simulink model "VITM"  (R2017b)
settings: Solver=FixedStepDiscrete  StartTime=0.0  StopTime=inf  FixedStep=vitk_stepSize  RelTol=1e-3  EnableMultiTasking=on
values from neighbouring files (symbols this model uses):
  vitc_CellPackVolTol = 12    [VITM_init.m]
  vitc_CellTempFaultTimer = 10    [VITM_init.m]
  vitc_CellTempFilterC = 1.0    (= 1)    [VITM_init.m]
  vitc_CellTempHighFaultReset = 0    [VITM_init.m]
  vitc_CellTempLowFaultReset = 0    [VITM_init.m]
  vitc_CellTempMax = 70    [VITM_init.m]
  vitc_CellTempMin = -40    [VITM_init.m]
  vitc_CellVolFilterC = 1    [VITM_init.m]
  vitc_CellVoltageFaultTimer = 2    [VITM_init.m]
  vitc_CellVoltageHighFaultReset = 0    [VITM_init.m]
  vitc_CellVoltageLowFaultReset = 0    [VITM_init.m]
  vitc_CellVoltageMax = 4.2    [VITM_init.m]
  vitc_CellVoltageMin = 2.7    [VITM_init.m]
  vitc_CoolantInletTFaultReset = 0    [VITM_init.m]
  vitc_CoolantInletTLowerLim = -40    [VITM_init.m]
  vitc_CoolantInletTUpperLim = 70    [VITM_init.m]
  vitc_CoolantOutletTFaultReset = 0    [VITM_init.m]
  vitc_CoolantOutletTLowerLim = -40    [VITM_init.m]
  vitc_CoolantOutletTUpperLim = 70    [VITM_init.m]
  vitc_CoolantTempFaultCounter = 5    [VITM_init.m]
  vitc_CoolantTFilterC = 0.9    [VITM_init.m]
  vitc_HVILFaultCounter = 1    [VITM_init.m]
  vitc_HVILFaultReset = 0    [VITM_init.m]
  vitc_PackCurFilterC = 1    [VITM_init.m]
  vitc_PackCurrentFaultReset = 0    [VITM_init.m]
  vitc_PackCurrentFaultTimer = 1    [VITM_init.m]
  vitc_PackCurrentLimit = 300    [VITM_init.m]
  vitc_PackVolFilterC = 1    [VITM_init.m]
  vitc_PackVoltageFaultReset = 0    [VITM_init.m]
  vitc_PackVoltageFaultTimer = 10    [VITM_init.m]
  vitc_VehVolFilterC = 1    [VITM_init.m]
  vitk_NumberInPara = 1    [VITM_init.m]
  vitk_NumberInSeries = 40    [VITM_init.m]
  vitk_stepSize = 0.1    [VITM_init.m]
libraries: simulink x1
settings Model: Creator=favv5g  LastModifiedBy=nctzv8
settings ConfigSet: Description=OpenECU configuration set for code generation under RTW-EC.
settings SolverCC: PositivePriorityOrder=on
settings DataIOCC: LimitDataPoints=on  SaveFormat=Array  SignalLogging=off  VisualizeSimOutput=off
settings OptimizationCC: DefaultParameterBehavior=Inlined  InlineInvariantSignals=on  ExpressionDepthLimit=2147483647  StateBitsets=on  DataBitsets=on  ZeroExternalMemoryAtStartup=off  ZeroInternalMemoryAtStartup=off  NoFixptDivByZeroProtection=on  EfficientFloat2IntCast=on  LifeSpan=1
settings DebuggingCC: SaveWithParameterizedLinksMsg=none  SignalResolutionControl=TryResolveAllWithWarning  MultiTaskDSMMsg=warning  MultiTaskCondExecSysMsg=none  SingleTaskRateTransMsg=error  CheckMatrixSingularityMsg=warning  VectorMatrixConversionMsg=warning  FcnCallInpInsideContextMsg=warning  SignalLabelMismatchMsg=warning  AllowSymbolicDim=off  StateNameClashWarn=warning  SFUnexpectedBacktrackingDiag=warning  SFNoUnconditionalDefaultTransitionDiag=warning  SFExecutionAtInitializationDiag=none
settings HardwareCC: ProdBitPerPointer=32  ProdBitPerSizeT=32  ProdBitPerPtrDiffT=32  ProdLargestAtomicInteger=Long  ProdLargestAtomicFloat=Double  ProdEndianess=BigEndian  ProdWordSize=32  ProdHWDeviceType=Freescale->32-bit PowerPC  TargetIntDivRoundTo=Zero  TargetEndianess=BigEndian  TargetHWDeviceType=Freescale->32-bit PowerPC  ProdEqTarget=off
settings ModelReferenceCC: PropagateSignalLabelsOutOfModel=off
settings SFSimCC: MATLABDynamicMemAlloc=off
settings RTWCC: SystemTargetFile=openecu_ert.tlc  MakeCommand=make_rtw optimized_floating_point=1  TemplateMakefile=openecu_ert_r2015b_64.tmf  Description=OpenECU Platform Target (ERT, optimised floating-point code)  RetainRTWFile=on  IncludeHyperlinkInReport=on
settings CodeAppCC: ForceParamTrailComments=on  IgnoreCustomStorageClasses=off  SimulinkDataObjDesc=on  CustomSymbolStrType=$N$R$M  InsertBlockDesc=on  StateflowObjectComments=on  InternalIdentifier=Classic
settings STFCustomTargetCC: TargetLibSuffix=.a  GenerateSampleERTMain=on  IncludeMdlTerminateFcn=off  CombineOutputUpdateFcns=on  IncludeFileDelimiter=UseQuote  ERTCustomFileBanners=on  SupportContinuousTime=off  RemoveResetFunc=on  MATLABClassNameForMDSCustomization=Simulink.SoftwareTarget.ERTCustomization  GRTInterface=off  SystemTargetFile=openecu_ert.tlc
settings ERTTargetCC: MultiwordLength=2048  GenerateSampleERTMain=on  ParMdlRefBuildCompliant=off  CompOptLevelCompliant=off  ConcurrentExecutionCompliant=off  IncludeMdlTerminateFcn=off  IncludeFileDelimiter=UseQuote  SupportNonInlinedSFcns=on  ModelStepFunctionPrototypeControlCompliant=off  CPPClassGenCompliant=off  UseToolchainInfoCompliant=off  ExtModeMexFile=noextcomm  InlinedParameterPlacement=NonHierarchical  ERTSrcFileBannerTemplate=oe_code_c_template.cgt  ERTHdrFileBannerTemplate=oe_code_h_template.cgt  ERTDataSrcFileTemplate=oe_data_c_template.cgt  ERTDataHdrFileTemplate=oe_data_h_template.cgt  ERTCustomFileTemplate=example_file_process.tlc  GlobalDataDefinition=InSeparateSourceFile  GlobalDataReference=InSeparateHeaderFile  ConvertIfToSwitch=off  SuppressUnreachableDefaultCases=off  EnableUserReplacementTypes=on
settings ConfigComp: CovMetricSettings=dw  CovHtmlReporting=on  CovSaveCumulativeToWorkspaceVar=on  CovSaveSingleToWorkspaceVar=on  CovExternalEMLEnable=off

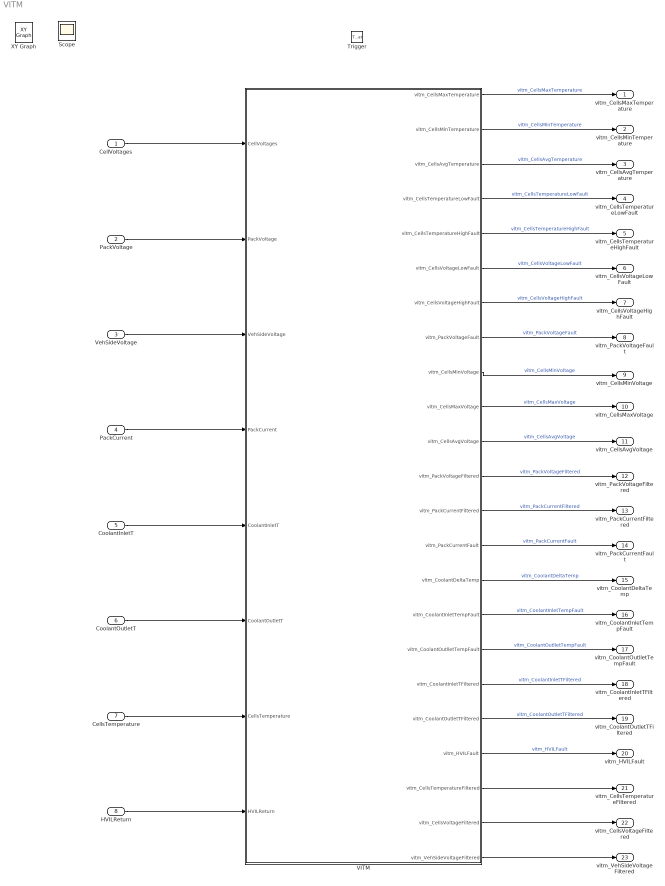
== system VITM ==
  CellVoltages : Inport  PortDimensions=40
  PackVoltage : Inport  Port=2
  VehSideVoltage : Inport  Port=3
  PackCurrent : Inport  Port=4
  CoolantInletT : Inport  Port=5
  CoolantOutletT : Inport  Port=6
  CellsTemperature : Inport  Port=7  PortDimensions=40
  HVILReturn : Inport  Port=8
  Trigger : TriggerPort  TriggerType=function-call  VariantControl=(inherit)  PortDimensions=1
  VITM : Subsystem  TreatAsAtomicUnit=on
  vitm_CellsMaxTemperature : Outport
  vitm_CellsMinTemperature : Outport  Port=2
  vitm_CellsAvgTemperature : Outport  Port=3
  vitm_CellsTemperatureLowFault : Outport  Port=4
  vitm_CellsTemperatureHighFault : Outport  Port=5
  vitm_CellsVoltageLowFault : Outport  Port=6
  vitm_CellsVoltageHighFault : Outport  Port=7
  vitm_PackVoltageFault : Outport  Port=8
  vitm_CellsMinVoltage : Outport  Port=9
  vitm_CellsMaxVoltage : Outport  Port=10
  vitm_CellsAvgVoltage : Outport  Port=11
  vitm_PackVoltageFiltered : Outport  Port=12
  vitm_PackCurrentFiltered : Outport  Port=13
  vitm_PackCurrentFault : Outport  Port=14
  vitm_CoolantDeltaTemp : Outport  Port=15
  vitm_CoolantInletTempFault : Outport  Port=16
  vitm_CoolantOutlletTempFault : Outport  Port=17
  vitm_CoolantInletTFiltered : Outport  Port=18
  vitm_CoolantOutletTFiltered : Outport  Port=19
  vitm_HVILFault : Outport  Port=20
  vitm_CellsTemperatureFiltered : Outport  Port=21
  vitm_CellsVoltageFiltered : Outport  Port=22  PortDimensions=40
  vitm_VehSideVoltageFiltered : Outport  Port=23
  Scope : Scope
  XY Graph : simulink/Sinks/XY Graph  IOType=viewer  xmin=-1  xmax=1  ymin=-1  ymax=1  st=-1
  wires:
  CellVoltages/1 -> VITM/1(CellVoltages)
  PackVoltage/1 -> VITM/2(PackVoltage)
  VehSideVoltage/1 -> VITM/3(VehSideVoltage)
  PackCurrent/1 -> VITM/4(PackCurrent)
  CoolantInletT/1 -> VITM/5(CoolantInletT)
  CoolantOutletT/1 -> VITM/6(CoolantOutletT)
  CellsTemperature/1 -> VITM/7(CellsTemperature)
  VITM/2(vitm_CellsMinTemperature) -> vitm_CellsMinTemperature/1  "vitm_CellsMinTemperature"
  VITM/3(vitm_CellsAvgTemperature) -> vitm_CellsAvgTemperature/1  "vitm_CellsAvgTemperature"
  VITM/1(vitm_CellsMaxTemperature) -> vitm_CellsMaxTemperature/1  "vitm_CellsMaxTemperature"
  VITM/4(vitm_CellsTemperatureLowFault) -> vitm_CellsTemperatureLowFault/1  "vitm_CellsTemperatureLowFault"
  VITM/6(vitm_CellsVoltageLowFault) -> vitm_CellsVoltageLowFault/1  "vitm_CellsVoltageLowFault"
  VITM/7(vitm_CellsVoltageHighFault) -> vitm_CellsVoltageHighFault/1  "vitm_CellsVoltageHighFault"
  VITM/5(vitm_CellsTemperatureHighFault) -> vitm_CellsTemperatureHighFault/1  "vitm_CellsTemperatureHighFault"
  VITM/9(vitm_CellsMinVoltage) -> vitm_CellsMinVoltage/1  "vitm_CellsMinVoltage"
  VITM/8(vitm_PackVoltageFault) -> vitm_PackVoltageFault/1  "vitm_PackVoltageFault"
  VITM/18(vitm_CoolantInletTFiltered) -> vitm_CoolantInletTFiltered/1  "vitm_CoolantInletTFiltered"
  VITM/10(vitm_CellsMaxVoltage) -> vitm_CellsMaxVoltage/1  "vitm_CellsMaxVoltage"
  VITM/12(vitm_PackVoltageFiltered) -> vitm_PackVoltageFiltered/1  "vitm_PackVoltageFiltered"
  VITM/14(vitm_PackCurrentFault) -> vitm_PackCurrentFault/1  "vitm_PackCurrentFault"
  VITM/15(vitm_CoolantDeltaTemp) -> vitm_CoolantDeltaTemp/1  "vitm_CoolantDeltaTemp"
  VITM/13(vitm_PackCurrentFiltered) -> vitm_PackCurrentFiltered/1  "vitm_PackCurrentFiltered"
  VITM/11(vitm_CellsAvgVoltage) -> vitm_CellsAvgVoltage/1  "vitm_CellsAvgVoltage"
  VITM/16(vitm_CoolantInletTempFault) -> vitm_CoolantInletTempFault/1  "vitm_CoolantInletTempFault"
  VITM/17(vitm_CoolantOutlletTempFault) -> vitm_CoolantOutlletTempFault/1  "vitm_CoolantOutlletTempFault"
  VITM/19(vitm_CoolantOutletTFiltered) -> vitm_CoolantOutletTFiltered/1  "vitm_CoolantOutletTFiltered"
  HVILReturn/1 -> VITM/8(HVILReturn)
  VITM/23(vitm_VehSideVoltageFiltered) -> vitm_VehSideVoltageFiltered/1
  VITM/22(vitm_CellsVoltageFiltered) -> vitm_CellsVoltageFiltered/1
  VITM/21(vitm_CellsTemperatureFiltered) -> vitm_CellsTemperatureFiltered/1
  VITM/20(vitm_HVILFault) -> vitm_HVILFault/1  "vitm_HVILFault"

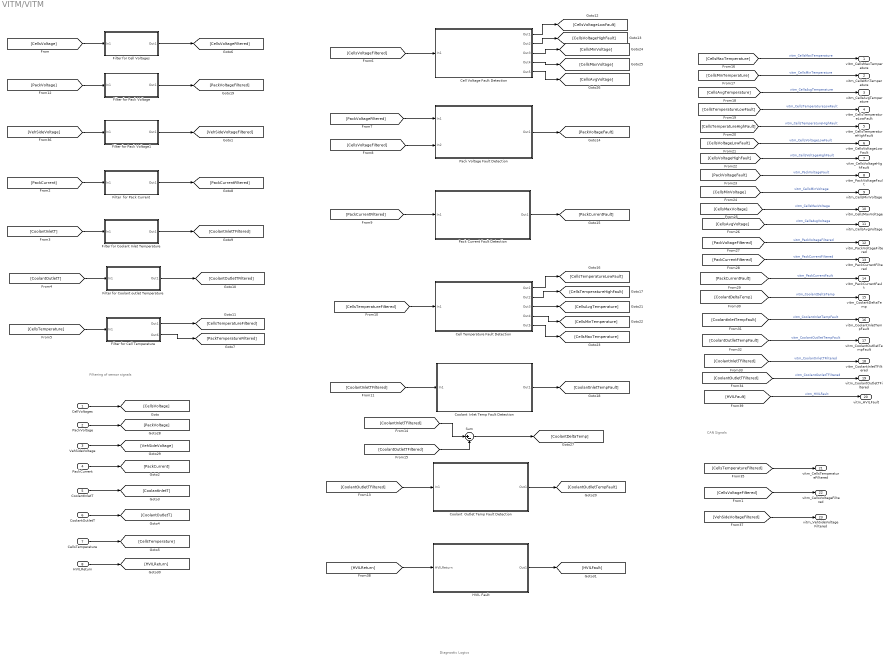
== system VITM/VITM ==
  note: Diagnostic Logics
  note: Filtering of sensor signals
  note: CAN Signals
  CellVoltages : Inport  PortDimensions=40
  PackVoltage : Inport  Port=2
  VehSideVoltage : Inport  Port=3
  PackCurrent : Inport  Port=4
  CoolantInletT : Inport  Port=5
  CoolantOutletT : Inport  Port=6
  CellsTemperature : Inport  Port=7  PortDimensions=40
  HVILReturn : Inport  Port=8
  " Filter for Cell Voltages" : Subsystem
  " Filter for Pack Voltage" : Subsystem
  " Filter for Pack Voltage1" : Subsystem
  Cell Temperature Fault Detection : Subsystem
  Cell Voltage Fault Detection : Subsystem
  Coolant  Inlet Temp Fault Detection : Subsystem
  Coolant  Outlet Temp Fault Detection : Subsystem
  Filter  for Pack Current : Subsystem
  Filter for Cell Temperature : Subsystem
  Filter for Coolant Inlet Temperature : Subsystem
  Filter for Coolant outlet Temperature : Subsystem
  HVIL Fault : Subsystem
  Pack Current Fault Detection : Subsystem
  Pack Voltage Fault Detection : Subsystem
  Sum : Sum  Inputs=|+-
  vitm_CellsMaxTemperature : Outport
  vitm_CellsMinTemperature : Outport  Port=2
  vitm_CellsAvgTemperature : Outport  Port=3
  vitm_CellsTemperatureLowFault : Outport  Port=4
  vitm_CellsTemperatureHighFault : Outport  Port=5
  vitm_CellsVoltageLowFault : Outport  Port=6
  vitm_CellsVoltageHighFault : Outport  Port=7
  vitm_PackVoltageFault : Outport  Port=8
  vitm_CellsMinVoltage : Outport  Port=9
  vitm_CellsMaxVoltage : Outport  Port=10
  vitm_CellsAvgVoltage : Outport  Port=11
  vitm_PackVoltageFiltered : Outport  Port=12
  vitm_PackCurrentFiltered : Outport  Port=13
  vitm_PackCurrentFault : Outport  Port=14
  vitm_CoolantDeltaTemp : Outport  Port=15
  vitm_CoolantInletTempFault : Outport  Port=16
  vitm_CoolantOutlletTempFault : Outport  Port=17
  vitm_CoolantInletTFiltered : Outport  Port=18
  vitm_CoolantOutletTFiltered : Outport  Port=19
  vitm_HVILFault : Outport  Port=20
  vitm_CellsTemperatureFiltered : Outport  Port=21
  vitm_CellsVoltageFiltered : Outport  Port=22
  vitm_VehSideVoltageFiltered : Outport  Port=23
  wires:
  [VehSideVoltage] -> " Filter for Pack Voltage1"/1(In1)
  VehSideVoltage/1 -> [VehSideVoltage]
  " Filter for Pack Voltage1"/1(Out1) -> [VehSideVoltageFiltered]
  [VehSideVoltageFiltered] -> vitm_VehSideVoltageFiltered/1
  [PackVoltage] -> " Filter for Pack Voltage"/1(In1)
  PackVoltage/1 -> [PackVoltage]
  " Filter for Pack Voltage"/1(Out1) -> [PackVoltageFiltered]
  CoolantOutletT/1 -> [CoolantOutletT]
  Filter  for Pack Current/1(Out1) -> [PackCurrentFiltered]
  [CoolantInletT] -> Filter for Coolant Inlet Temperature/1(In1)
  Filter for Coolant Inlet Temperature/1(Out1) -> [CoolantInletTFiltered]
  [CellsVoltage] -> " Filter for Cell Voltages"/1(In1)
  CellVoltages/1 -> [CellsVoltage]
  PackCurrent/1 -> [PackCurrent]
  CellsTemperature/1 -> [CellsTemperature]
  CoolantInletT/1 -> [CoolantInletT]
  " Filter for Cell Voltages"/1(Out1) -> [CellsVoltageFiltered]
  [PackCurrent] -> Filter  for Pack Current/1(In1)
  Cell Voltage Fault Detection/2(Out2) -> [CellsVoltageHighFault]
  Pack Current Fault Detection/1(Out1) -> [PackCurrentFault]
  [CoolantOutletT] -> Filter for Coolant outlet Temperature/1(In1)
  [CellsTemperatureFiltered] -> Cell Temperature Fault Detection/1(In1)
  Cell Temperature Fault Detection/2(Out2) -> [CellsTemperatureHighFault]
  Coolant  Inlet Temp Fault Detection/1(Out1) -> [CoolantInletTempFault]
  [CellsTemperature] -> Filter for Cell Temperature/1(In1)
  [PackVoltageFiltered] -> Pack Voltage Fault Detection/1(In1)
  Cell Temperature Fault Detection/1(Out1) -> [CellsTemperatureLowFault]
  Cell Voltage Fault Detection/1(Out1) -> [CellsVoltageLowFault]
  Cell Temperature Fault Detection/5(Out5) -> [CellsMaxTemperature]
  Cell Temperature Fault Detection/4(Out4) -> [CellsMinTemperature]
  Cell Voltage Fault Detection/3(Out3) -> [CellsMinVoltage]
  [CellsVoltageFiltered] -> Pack Voltage Fault Detection/2(In2)
  Cell Voltage Fault Detection/4(Out4) -> [CellsMaxVoltage]
  [CoolantInletTFiltered] -> Sum/1
  [CellsVoltageFiltered] -> Cell Voltage Fault Detection/1(In1)
  [PackCurrentFiltered] -> Pack Current Fault Detection/1(In1)
  [CoolantOutletTFiltered] -> Sum/2
  Sum/1 -> [CoolantDeltaTemp]
  [CellsMinTemperature] -> vitm_CellsMinTemperature/1  "vitm_CellsMinTemperature"
  [CoolantInletTFiltered] -> Coolant  Inlet Temp Fault Detection/1(In1)
  [CellsAvgTemperature] -> vitm_CellsAvgTemperature/1  "vitm_CellsAvgTemperature"
  Coolant  Outlet Temp Fault Detection/1(Out1) -> [CoolantOutlletTempFault]
  [CoolantOutletTFiltered] -> Coolant  Outlet Temp Fault Detection/1(In1)
  Cell Voltage Fault Detection/5(Out5) -> [CellsAvgVoltage]
  Cell Temperature Fault Detection/3(Out3) -> [CellsAvgTemperature]
  [CellsMaxTemperature] -> vitm_CellsMaxTemperature/1  "vitm_CellsMaxTemperature"
  Filter for Cell Temperature/1(Out1) -> [CellsTemperatureFiltered]
  Filter for Coolant outlet Temperature/1(Out1) -> [CoolantOutletTFiltered]
  Pack Voltage Fault Detection/1(Out1) -> [PackVoltageFault]
  [CellsTemperatureLowFault] -> vitm_CellsTemperatureLowFault/1  "vitm_CellsTemperatureLowFault"
  [CellsVoltageLowFault] -> vitm_CellsVoltageLowFault/1  "vitm_CellsVoltageLowFault"
  [CellsVoltageHighFault] -> vitm_CellsVoltageHighFault/1  "vitm_CellsVoltageHighFault"
  [CellsTemperatureHighFault] -> vitm_CellsTemperatureHighFault/1  "vitm_CellsTemperatureHighFault"
  [CellsMinVoltage] -> vitm_CellsMinVoltage/1  "vitm_CellsMinVoltage"
  [PackVoltageFault] -> vitm_PackVoltageFault/1  "vitm_PackVoltageFault"
  [CoolantInletTFiltered] -> vitm_CoolantInletTFiltered/1  "vitm_CoolantInletTFiltered"
  [CellsMaxVoltage] -> vitm_CellsMaxVoltage/1  "vitm_CellsMaxVoltage"
  [PackVoltageFiltered] -> vitm_PackVoltageFiltered/1  "vitm_PackVoltageFiltered"
  [PackCurrentFault] -> vitm_PackCurrentFault/1  "vitm_PackCurrentFault"
  [CoolantDeltaTemp] -> vitm_CoolantDeltaTemp/1  "vitm_CoolantDeltaTemp"
  [PackCurrentFiltered] -> vitm_PackCurrentFiltered/1  "vitm_PackCurrentFiltered"
  [CellsAvgVoltage] -> vitm_CellsAvgVoltage/1  "vitm_CellsAvgVoltage"
  [CoolantInletTempFault] -> vitm_CoolantInletTempFault/1  "vitm_CoolantInletTempFault"
  [CoolantOutlletTempFault] -> vitm_CoolantOutlletTempFault/1  "vitm_CoolantOutlletTempFault"
  [CoolantOutletTFiltered] -> vitm_CoolantOutletTFiltered/1  "vitm_CoolantOutletTFiltered"
  Filter for Cell Temperature/2(Out6) -> [PackTemperatureFiltered]
  [CellsTemperatureFiltered] -> vitm_CellsTemperatureFiltered/1
  [CellsVoltageFiltered] -> vitm_CellsVoltageFiltered/1
  HVILReturn/1 -> [HVILReturn]
  HVIL Fault/1(Out1) -> [HVILFault]
  [HVILReturn] -> HVIL Fault/1(HVILReturn)
  [HVILFault] -> vitm_HVILFault/1  "vitm_HVILFault"

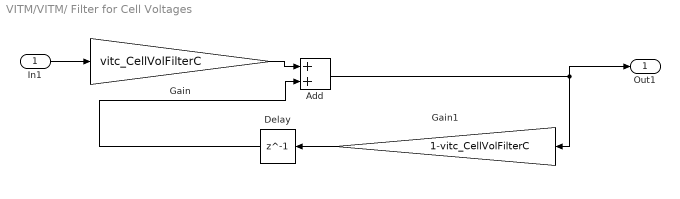
== system VITM/VITM/ Filter for Cell Voltages ==
  In1 : Inport
  Add : Sum
  Delay : Delay  DelayLength=1
  Gain : Gain  Gain=vitc_CellVolFilterC
  Gain1 : Gain  Gain=1-vitc_CellVolFilterC
  Out1 : Outport
  wires:
  Add/1 -> Out1/1, Gain1/1
  Gain1/1 -> Delay/1
  Delay/1 -> Add/2
  In1/1 -> Gain/1
  Gain/1 -> Add/1

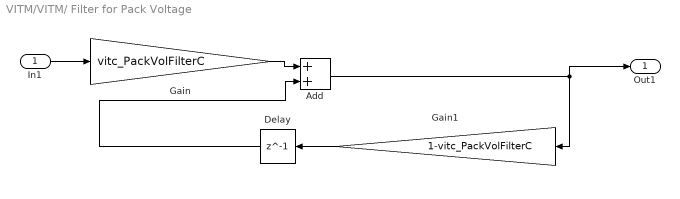
== system VITM/VITM/ Filter for Pack Voltage ==
  In1 : Inport
  Add : Sum
  Delay : Delay  DelayLength=1
  Gain : Gain  Gain=vitc_PackVolFilterC
  Gain1 : Gain  Gain=1-vitc_PackVolFilterC
  Out1 : Outport
  wires:
  Add/1 -> Out1/1, Gain1/1
  Gain1/1 -> Delay/1
  Delay/1 -> Add/2
  In1/1 -> Gain/1
  Gain/1 -> Add/1

== system VITM/VITM/ Filter for Pack Voltage1 ==
  In1 : Inport
  Add : Sum
  Delay : Delay  DelayLength=1
  Gain : Gain  Gain=vitc_VehVolFilterC
  Gain1 : Gain  Gain=1-vitc_VehVolFilterC
  Out1 : Outport
  wires:
  Add/1 -> Out1/1, Gain1/1
  Gain1/1 -> Delay/1
  Delay/1 -> Add/2
  In1/1 -> Gain/1
  Gain/1 -> Add/1

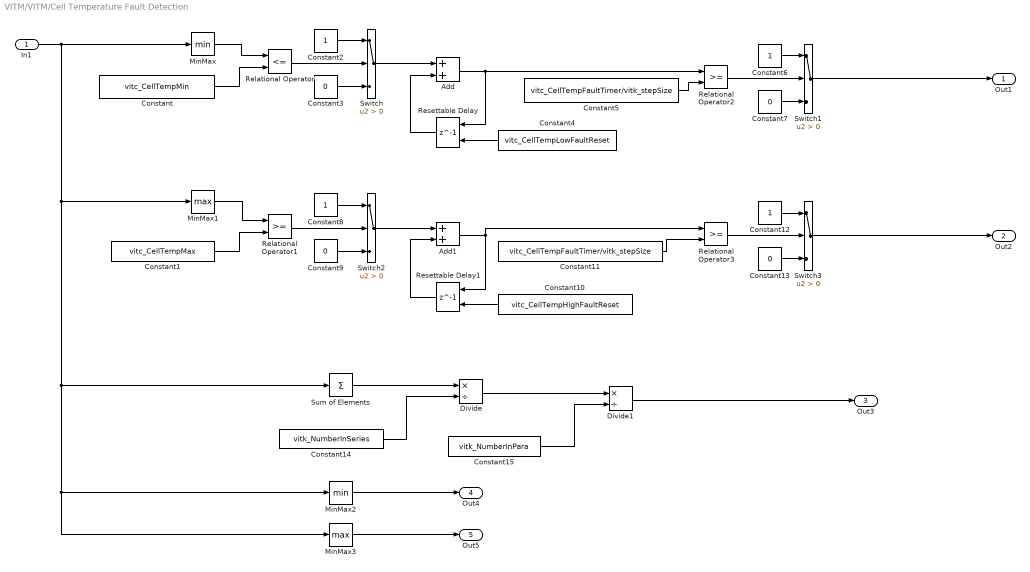
== system VITM/VITM/Cell Temperature Fault Detection ==
  In1 : Inport
  Add : Sum
  Add1 : Sum
  Constant : Constant  Value=vitc_CellTempMin
  Constant1 : Constant  Value=vitc_CellTempMax
  Constant10 : Constant  Value=vitc_CellTempHighFaultReset
  Constant11 : Constant  Value=vitc_CellTempFaultTimer/vitk_stepSize
  Constant12 : Constant  OutDataTypeStr=uint8
  Constant13 : Constant  Value=0  OutDataTypeStr=uint8
  Constant14 : Constant  Value=vitk_NumberInSeries
  Constant15 : Constant  Value=vitk_NumberInPara
  Constant2 : Constant
  Constant3 : Constant  Value=0
  Constant4 : Constant  Value=vitc_CellTempLowFaultReset
  Constant5 : Constant  Value=vitc_CellTempFaultTimer/vitk_stepSize
  Constant6 : Constant  OutDataTypeStr=uint8
  Constant7 : Constant  Value=0  OutDataTypeStr=uint8
  Constant8 : Constant
  Constant9 : Constant  Value=0
  Divide : Product  Inputs=*/
  Divide1 : Product  Inputs=*/
  MinMax : MinMax
  MinMax1 : MinMax  Function=max
  MinMax2 : MinMax
  MinMax3 : MinMax  Function=max
  Relational Operator : RelationalOperator  Operator=<=  OutDataTypeStr=boolean  RndMeth=Nearest
  Relational Operator1 : RelationalOperator  OutDataTypeStr=boolean  RndMeth=Nearest
  Relational Operator2 : RelationalOperator  OutDataTypeStr=boolean  RndMeth=Nearest
  Relational Operator3 : RelationalOperator  OutDataTypeStr=boolean  RndMeth=Nearest
  Resettable Delay : Delay  DelayLength=1  ExternalReset=Rising
      settings: InputPortMap=u0,r5
  Resettable Delay1 : Delay  DelayLength=1  ExternalReset=Rising
      settings: InputPortMap=u0,r5
  Sum of Elements : Sum  Inputs=+
  Switch{,1..3} (4 alike) : Switch  Criteria=u2 > Threshold
  Out1 : Outport
  Out2 : Outport  Port=2
  Out3 : Outport  Port=3
  Out4 : Outport  Port=4
  Out5 : Outport  Port=5
  wires:
  Constant4/1 -> Resettable Delay/2
  Constant3/1 -> Switch/3
  Relational Operator/1 -> Switch/2
  Relational Operator2/1 -> Switch1/2
  Constant2/1 -> Switch/1
  Constant6/1 -> Switch1/1
  Constant7/1 -> Switch1/3
  MinMax/1 -> Relational Operator/1
  Constant/1 -> Relational Operator/2
  MinMax1/1 -> Relational Operator1/1
  Constant1/1 -> Relational Operator1/2
  Switch3/1 -> Out2/1
  Switch1/1 -> Out1/1
  Switch/1 -> Add/1
  Add/1 -> Relational Operator2/1, Resettable Delay/1
  Constant5/1 -> Relational Operator2/2
  Resettable Delay/1 -> Add/2
  Add1/1 -> Relational Operator3/1, Resettable Delay1/1
  Constant9/1 -> Switch2/3
  Constant8/1 -> Switch2/1
  Constant11/1 -> Relational Operator3/2
  Constant10/1 -> Resettable Delay1/2
  Constant13/1 -> Switch3/3
  Constant12/1 -> Switch3/1
  Switch2/1 -> Add1/1
  Relational Operator3/1 -> Switch3/2
  Relational Operator1/1 -> Switch2/2
  Resettable Delay1/1 -> Add1/2
  In1/1 -> MinMax/1, MinMax1/1, Sum of Elements/1, MinMax2/1, MinMax3/1
  Sum of Elements/1 -> Divide/1
  Constant14/1 -> Divide/2
  Divide/1 -> Divide1/1
  Constant15/1 -> Divide1/2
  Divide1/1 -> Out3/1
  MinMax2/1 -> Out4/1
  MinMax3/1 -> Out5/1

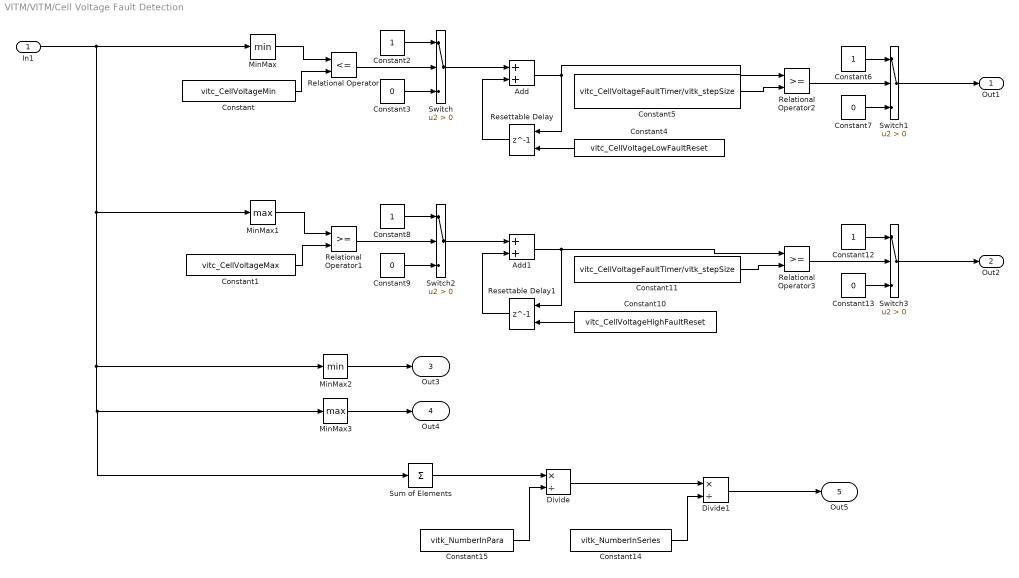
== system VITM/VITM/Cell Voltage Fault Detection ==
  In1 : Inport
  Add : Sum
  Add1 : Sum
  Constant : Constant  Value=vitc_CellVoltageMin
  Constant1 : Constant  Value=vitc_CellVoltageMax
  Constant10 : Constant  Value=vitc_CellVoltageHighFaultReset
  Constant11 : Constant  Value=vitc_CellVoltageFaultTimer/vitk_stepSize
  Constant12 : Constant  OutDataTypeStr=uint8
  Constant13 : Constant  Value=0  OutDataTypeStr=uint8
  Constant14 : Constant  Value=vitk_NumberInSeries
  Constant15 : Constant  Value=vitk_NumberInPara
  Constant2 : Constant
  Constant3 : Constant  Value=0
  Constant4 : Constant  Value=vitc_CellVoltageLowFaultReset
  Constant5 : Constant  Value=vitc_CellVoltageFaultTimer/vitk_stepSize
  Constant6 : Constant  OutDataTypeStr=uint8
  Constant7 : Constant  Value=0  OutDataTypeStr=uint8
  Constant8 : Constant
  Constant9 : Constant  Value=0
  Divide : Product  Inputs=*/
  Divide1 : Product  Inputs=*/  OutDataTypeStr=double
  MinMax : MinMax
  MinMax1 : MinMax  Function=max
  MinMax2 : MinMax
  MinMax3 : MinMax  Function=max
  Relational Operator : RelationalOperator  Operator=<=  OutDataTypeStr=boolean  RndMeth=Nearest
  Relational Operator1 : RelationalOperator  OutDataTypeStr=boolean  RndMeth=Nearest
  Relational Operator2 : RelationalOperator  OutDataTypeStr=boolean  RndMeth=Nearest
  Relational Operator3 : RelationalOperator  OutDataTypeStr=boolean  RndMeth=Nearest
  Resettable Delay : Delay  DelayLength=1  ExternalReset=Rising
      settings: InputPortMap=u0,r5
  Resettable Delay1 : Delay  DelayLength=1  ExternalReset=Rising
      settings: InputPortMap=u0,r5
  Sum of Elements : Sum  Inputs=+
  Switch{,1..3} (4 alike) : Switch  Criteria=u2 > Threshold
  Out1 : Outport
  Out2 : Outport  Port=2
  Out3 : Outport  Port=3
  Out4 : Outport  Port=4
  Out5 : Outport  Port=5  OutDataTypeStr=double
  wires:
  Constant4/1 -> Resettable Delay/2
  Constant3/1 -> Switch/3
  Relational Operator/1 -> Switch/2
  Relational Operator2/1 -> Switch1/2
  Constant2/1 -> Switch/1
  Constant6/1 -> Switch1/1
  Constant7/1 -> Switch1/3
  MinMax/1 -> Relational Operator/1
  Constant/1 -> Relational Operator/2
  MinMax1/1 -> Relational Operator1/1
  Constant1/1 -> Relational Operator1/2
  Switch3/1 -> Out2/1
  Switch1/1 -> Out1/1
  Switch/1 -> Add/1
  Add/1 -> Relational Operator2/1, Resettable Delay/1
  Constant5/1 -> Relational Operator2/2
  Resettable Delay/1 -> Add/2
  Add1/1 -> Relational Operator3/1, Resettable Delay1/1
  Constant9/1 -> Switch2/3
  Constant8/1 -> Switch2/1
  Constant11/1 -> Relational Operator3/2
  Constant10/1 -> Resettable Delay1/2
  Constant13/1 -> Switch3/3
  Constant12/1 -> Switch3/1
  Switch2/1 -> Add1/1
  Relational Operator3/1 -> Switch3/2
  Relational Operator1/1 -> Switch2/2
  Resettable Delay1/1 -> Add1/2
  MinMax2/1 -> Out3/1
  MinMax3/1 -> Out4/1
  In1/1 -> MinMax/1, MinMax1/1, MinMax2/1, MinMax3/1, Sum of Elements/1
  Sum of Elements/1 -> Divide/1
  Divide/1 -> Divide1/1
  Divide1/1 -> Out5/1
  Constant15/1 -> Divide/2
  Constant14/1 -> Divide1/2

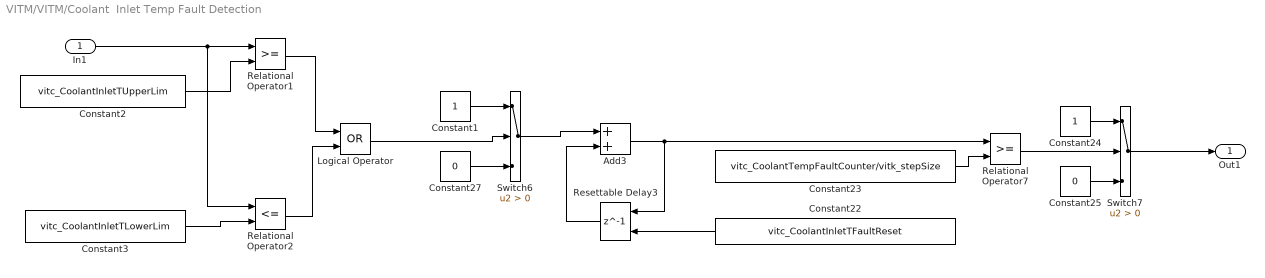
== system VITM/VITM/Coolant  Inlet Temp Fault Detection ==
  In1 : Inport
  Add3 : Sum
  Constant1 : Constant
  Constant2 : Constant  Value=vitc_CoolantInletTUpperLim
  Constant22 : Constant  Value=vitc_CoolantInletTFaultReset
  Constant23 : Constant  Value=vitc_CoolantTempFaultCounter/vitk_stepSize
  Constant24 : Constant  OutDataTypeStr=uint8
  Constant25 : Constant  Value=0  OutDataTypeStr=uint8
  Constant27 : Constant  Value=0
  Constant3 : Constant  Value=vitc_CoolantInletTLowerLim
  Logical Operator : Logic  Operator=OR  AllPortsSameDT=off  OutDataTypeStr=boolean
  Relational Operator1 : RelationalOperator  OutDataTypeStr=boolean  RndMeth=Nearest
  Relational Operator2 : RelationalOperator  Operator=<=  OutDataTypeStr=boolean  RndMeth=Nearest
  Relational Operator7 : RelationalOperator  OutDataTypeStr=boolean  RndMeth=Nearest
  Resettable Delay3 : Delay  DelayLength=1  ExternalReset=Rising
      settings: InputPortMap=u0,r5
  Switch6 : Switch  Criteria=u2 > Threshold
  Switch7 : Switch  Criteria=u2 > Threshold
  Out1 : Outport
  wires:
  Constant25/1 -> Switch7/3
  Constant27/1 -> Switch6/3
  Constant23/1 -> Relational Operator7/2
  Switch6/1 -> Add3/1
  Constant1/1 -> Switch6/1
  Constant24/1 -> Switch7/1
  Constant22/1 -> Resettable Delay3/2
  Add3/1 -> Relational Operator7/1, Resettable Delay3/1
  Resettable Delay3/1 -> Add3/2
  Switch7/1 -> Out1/1
  Relational Operator7/1 -> Switch7/2
  Constant2/1 -> Relational Operator1/2
  Constant3/1 -> Relational Operator2/2
  Relational Operator1/1 -> Logical Operator/1
  Relational Operator2/1 -> Logical Operator/2
  Logical Operator/1 -> Switch6/2
  In1/1 -> Relational Operator2/1, Relational Operator1/1

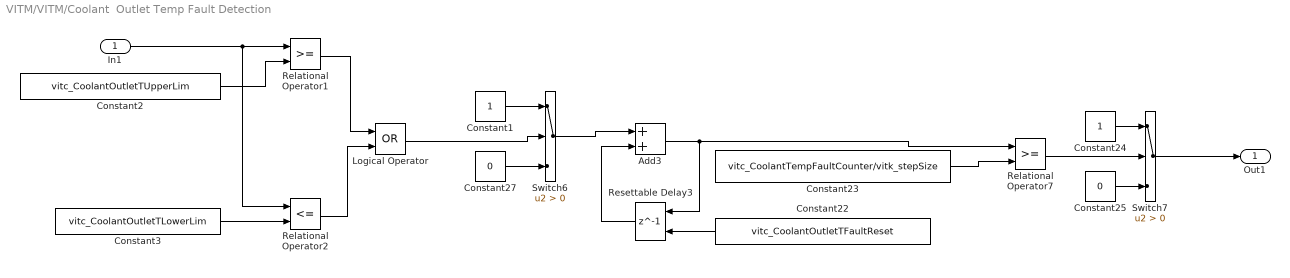
== system VITM/VITM/Coolant  Outlet Temp Fault Detection ==
  In1 : Inport
  Add3 : Sum
  Constant1 : Constant
  Constant2 : Constant  Value=vitc_CoolantOutletTUpperLim
  Constant22 : Constant  Value=vitc_CoolantOutletTFaultReset
  Constant23 : Constant  Value=vitc_CoolantTempFaultCounter/vitk_stepSize
  Constant24 : Constant  OutDataTypeStr=uint8
  Constant25 : Constant  Value=0  OutDataTypeStr=uint8
  Constant27 : Constant  Value=0
  Constant3 : Constant  Value=vitc_CoolantOutletTLowerLim
  Logical Operator : Logic  Operator=OR  AllPortsSameDT=off  OutDataTypeStr=boolean
  Relational Operator1 : RelationalOperator  OutDataTypeStr=boolean  RndMeth=Nearest
  Relational Operator2 : RelationalOperator  Operator=<=  OutDataTypeStr=boolean  RndMeth=Nearest
  Relational Operator7 : RelationalOperator  OutDataTypeStr=boolean  RndMeth=Nearest
  Resettable Delay3 : Delay  DelayLength=1  ExternalReset=Rising
      settings: InputPortMap=u0,r5
  Switch6 : Switch  Criteria=u2 > Threshold
  Switch7 : Switch  Criteria=u2 > Threshold
  Out1 : Outport
  wires:
  Constant25/1 -> Switch7/3
  Constant27/1 -> Switch6/3
  Constant23/1 -> Relational Operator7/2
  Switch6/1 -> Add3/1
  Constant1/1 -> Switch6/1
  Constant24/1 -> Switch7/1
  Constant22/1 -> Resettable Delay3/2
  Add3/1 -> Relational Operator7/1, Resettable Delay3/1
  Resettable Delay3/1 -> Add3/2
  Switch7/1 -> Out1/1
  Relational Operator7/1 -> Switch7/2
  In1/1 -> Relational Operator2/1, Relational Operator1/1
  Constant2/1 -> Relational Operator1/2
  Constant3/1 -> Relational Operator2/2
  Relational Operator1/1 -> Logical Operator/1
  Relational Operator2/1 -> Logical Operator/2
  Logical Operator/1 -> Switch6/2

== system VITM/VITM/Filter  for Pack Current ==
  In1 : Inport
  Add1 : Sum
  Delay1 : Delay  DelayLength=1
  Gain2 : Gain  Gain=vitc_PackCurFilterC
  Gain3 : Gain  Gain=1-vitc_PackCurFilterC
  Out1 : Outport
  wires:
  Add1/1 -> Out1/1, Gain3/1
  Gain3/1 -> Delay1/1
  Delay1/1 -> Add1/2
  In1/1 -> Gain2/1
  Gain2/1 -> Add1/1

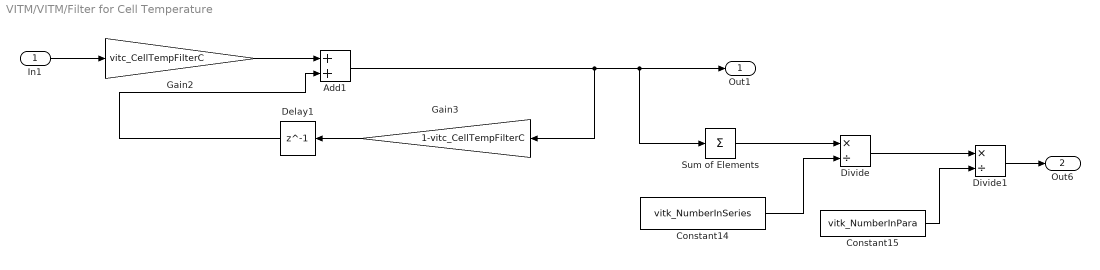
== system VITM/VITM/Filter for Cell Temperature ==
  In1 : Inport
  Add1 : Sum
  Constant14 : Constant  Value=vitk_NumberInSeries
  Constant15 : Constant  Value=vitk_NumberInPara
  Delay1 : Delay  DelayLength=1
  Divide : Product  Inputs=*/  OutDataTypeStr=double
  Divide1 : Product  Inputs=*/
  Gain2 : Gain  Gain=vitc_CellTempFilterC
  Gain3 : Gain  Gain=1-vitc_CellTempFilterC
  Sum of Elements : Sum  Inputs=+
  Out1 : Outport
  Out6 : Outport  Port=2
  wires:
  Add1/1 -> Sum of Elements/1, Out1/1, Gain3/1
  Gain3/1 -> Delay1/1
  Delay1/1 -> Add1/2
  In1/1 -> Gain2/1
  Gain2/1 -> Add1/1
  Sum of Elements/1 -> Divide/1
  Constant14/1 -> Divide/2
  Divide/1 -> Divide1/1
  Constant15/1 -> Divide1/2
  Divide1/1 -> Out6/1

== system VITM/VITM/Filter for Coolant Inlet Temperature ==
  In1 : Inport
  Add1 : Sum
  Delay1 : Delay  DelayLength=1
  Gain : Gain  Gain=vitc_CoolantTFilterC
  Gain1 : Gain  Gain=1-vitc_CoolantTFilterC
  Out1 : Outport
  wires:
  Add1/1 -> Out1/1, Gain1/1
  Gain1/1 -> Delay1/1
  Delay1/1 -> Add1/2
  In1/1 -> Gain/1
  Gain/1 -> Add1/1

== system VITM/VITM/Filter for Coolant outlet Temperature ==
  In1 : Inport
  Add1 : Sum
  Delay1 : Delay  DelayLength=1
  Gain : Gain  Gain=vitc_CoolantTFilterC
  Gain3 : Gain  Gain=1-vitc_CoolantTFilterC
  Out1 : Outport
  wires:
  Add1/1 -> Out1/1, Gain3/1
  Gain3/1 -> Delay1/1
  Delay1/1 -> Add1/2
  In1/1 -> Gain/1
  Gain/1 -> Add1/1

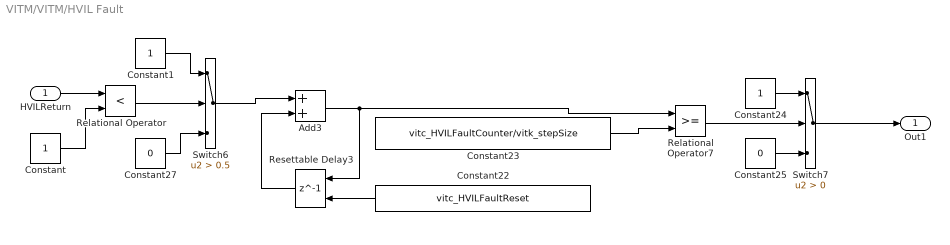
== system VITM/VITM/HVIL Fault ==
  HVILReturn : Inport
  Add3 : Sum
  Constant : Constant
  Constant1 : Constant
  Constant22 : Constant  Value=vitc_HVILFaultReset
  Constant23 : Constant  Value=vitc_HVILFaultCounter/vitk_stepSize
  Constant24 : Constant  OutDataTypeStr=uint8
  Constant25 : Constant  Value=0  OutDataTypeStr=uint8
  Constant27 : Constant  Value=0
  Relational Operator : RelationalOperator  Operator=<  OutDataTypeStr=boolean  RndMeth=Nearest
  Relational Operator7 : RelationalOperator  OutDataTypeStr=boolean  RndMeth=Nearest
  Resettable Delay3 : Delay  DelayLength=1  ExternalReset=Rising
      settings: InputPortMap=u0,r5
  Switch6 : Switch  Criteria=u2 > Threshold  Threshold=0.5
  Switch7 : Switch  Criteria=u2 > Threshold
  Out1 : Outport
  wires:
  Constant25/1 -> Switch7/3
  Constant27/1 -> Switch6/3
  Constant23/1 -> Relational Operator7/2
  Switch6/1 -> Add3/1
  Constant1/1 -> Switch6/1
  Constant24/1 -> Switch7/1
  Constant22/1 -> Resettable Delay3/2
  Add3/1 -> Relational Operator7/1, Resettable Delay3/1
  Resettable Delay3/1 -> Add3/2
  Switch7/1 -> Out1/1
  Relational Operator7/1 -> Switch7/2
  HVILReturn/1 -> Relational Operator/1
  Constant/1 -> Relational Operator/2
  Relational Operator/1 -> Switch6/2

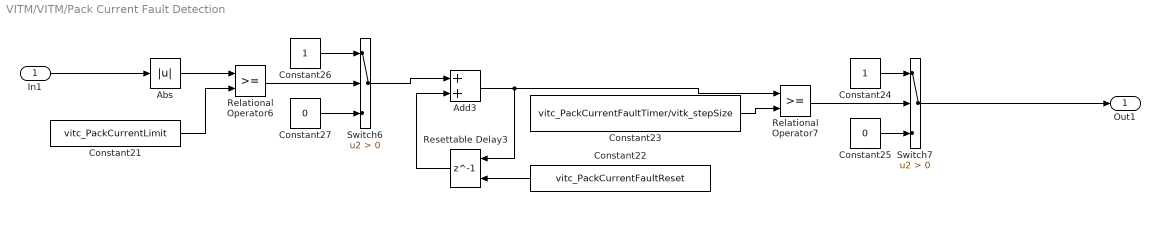
== system VITM/VITM/Pack Current Fault Detection ==
  In1 : Inport
  Abs : Abs
  Add3 : Sum
  Constant21 : Constant  Value=vitc_PackCurrentLimit
  Constant22 : Constant  Value=vitc_PackCurrentFaultReset
  Constant23 : Constant  Value=vitc_PackCurrentFaultTimer/vitk_stepSize
  Constant24 : Constant  OutDataTypeStr=uint8
  Constant25 : Constant  Value=0  OutDataTypeStr=uint8
  Constant26 : Constant
  Constant27 : Constant  Value=0
  Relational Operator6 : RelationalOperator  OutDataTypeStr=boolean  RndMeth=Nearest
  Relational Operator7 : RelationalOperator  OutDataTypeStr=boolean  RndMeth=Nearest
  Resettable Delay3 : Delay  DelayLength=1  ExternalReset=Rising
      settings: InputPortMap=u0,r5
  Switch6 : Switch  Criteria=u2 > Threshold
  Switch7 : Switch  Criteria=u2 > Threshold
  Out1 : Outport
  wires:
  Constant21/1 -> Relational Operator6/2
  Constant25/1 -> Switch7/3
  Constant27/1 -> Switch6/3
  Constant23/1 -> Relational Operator7/2
  Switch6/1 -> Add3/1
  Constant26/1 -> Switch6/1
  Constant24/1 -> Switch7/1
  Constant22/1 -> Resettable Delay3/2
  Add3/1 -> Relational Operator7/1, Resettable Delay3/1
  Resettable Delay3/1 -> Add3/2
  Switch7/1 -> Out1/1
  Relational Operator7/1 -> Switch7/2
  Relational Operator6/1 -> Switch6/2
  In1/1 -> Abs/1
  Abs/1 -> Relational Operator6/1

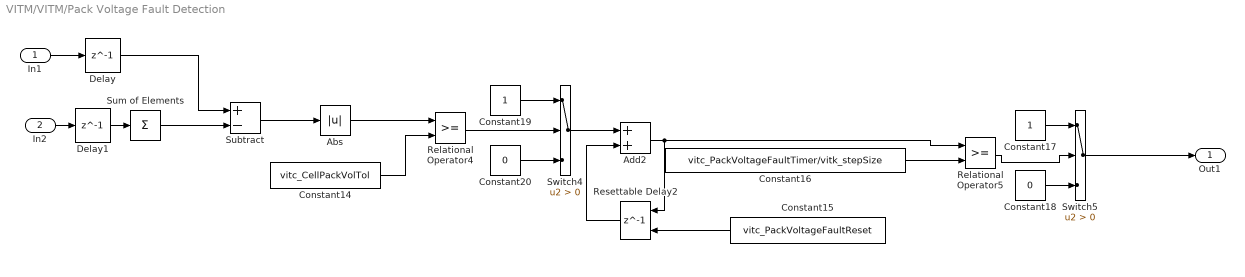
== system VITM/VITM/Pack Voltage Fault Detection ==
  In1 : Inport
  In2 : Inport  Port=2
  Abs : Abs
  Add2 : Sum
  Constant14 : Constant  Value=vitc_CellPackVolTol
  Constant15 : Constant  Value=vitc_PackVoltageFaultReset
  Constant16 : Constant  Value=vitc_PackVoltageFaultTimer/vitk_stepSize
  Constant17 : Constant  OutDataTypeStr=uint8
  Constant18 : Constant  Value=0  OutDataTypeStr=uint8
  Constant19 : Constant
  Constant20 : Constant  Value=0
  Delay : Delay  DelayLength=1
  Delay1 : Delay  DelayLength=1
  Relational Operator4 : RelationalOperator  OutDataTypeStr=boolean  RndMeth=Nearest
  Relational Operator5 : RelationalOperator  OutDataTypeStr=boolean  RndMeth=Nearest
  Resettable Delay2 : Delay  DelayLength=1  ExternalReset=Rising
      settings: InputPortMap=u0,r5
  Subtract : Sum  Inputs=+-
  Sum of Elements : Sum  Inputs=+
  Switch4 : Switch  Criteria=u2 > Threshold
  Switch5 : Switch  Criteria=u2 > Threshold
  Out1 : Outport
  wires:
  Sum of Elements/1 -> Subtract/2
  Subtract/1 -> Abs/1
  In1/1 -> Delay/1
  Constant20/1 -> Switch4/3
  Constant19/1 -> Switch4/1
  Add2/1 -> Relational Operator5/1, Resettable Delay2/1
  Constant15/1 -> Resettable Delay2/2
  Constant16/1 -> Relational Operator5/2
  Constant17/1 -> Switch5/1
  Constant18/1 -> Switch5/3
  Relational Operator4/1 -> Switch4/2
  Relational Operator5/1 -> Switch5/2
  Switch5/1 -> Out1/1
  Switch4/1 -> Add2/1
  Resettable Delay2/1 -> Add2/2
  In2/1 -> Delay1/1
  Abs/1 -> Relational Operator4/1
  Constant14/1 -> Relational Operator4/2
  Delay/1 -> Subtract/1
  Delay1/1 -> Sum of Elements/1
